simulink model "OcularMotorLabModel_2023_12_21_M21b"  (R2021b)
settings: Solver=FixedStepAuto  StartTime=tStart  StopTime=tFinal  FixedStep=0.001  RelTol=1e-3
undefined symbols (not defined in the file or in its folder): Asp, Asp1, Asp2, e0sp, gaussian, Gpc, GPos, Gsl, HeadToEye, IPD, psi, Psp1, RotFbk, SacThDeg, SatSp, sigbuilder_block, SomFbk, T1, T2, Tccanal, Tcn, Tcr, Tcsp, TCvs, tdm, tdsp1, tdsp2, tdsp3, tdv, Tsl, Tz, w
libraries: matrix_library x16, vrlib x9, simulink_extras x8, simulink x1
(part 1 of 2)
settings Model: Creator=raulr  LastModifiedBy=jom

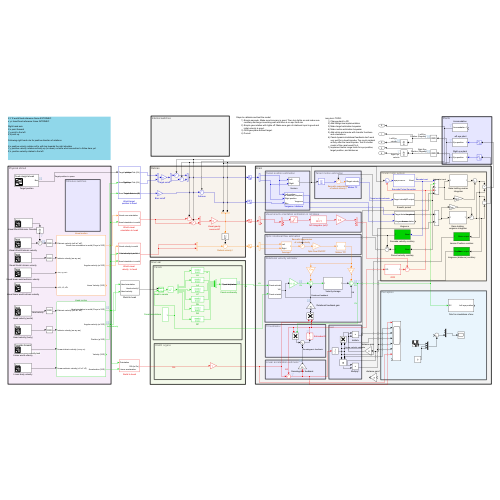
[thumbnail: Simulink's stored preview of the top-level diagram]
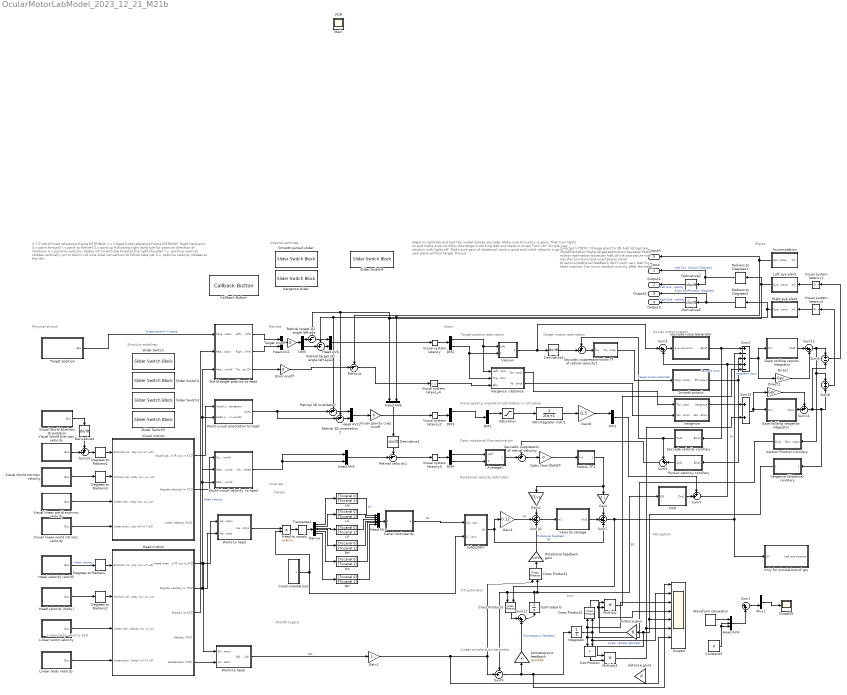
== system OcularMotorLabModel_2023_12_21_M21b ==
  note: Linear body velocity bad
  note: Internal switches
  note: Stimulus switches
  note: Plants
  note: Steps to calibrate and test the model
      | Simple saccade. Make sure Accuracy is good. Then turn lights on and make sure corollary discharge is working well and there is no spv from okn
      | Simple yaw rotation with lights off. Make sure gain of rotational input is good and initial velocity is good.
      | OKN yaw plane without target.
      | Pursuit
  note: X Y Z world fixed reference frame EXTRINSIC
      | x y z head fixed reference frame INTRINSIC
      |
      | Right hand axis
      | X,x point forward
      | Y,y point to the left
      | Z,z point up
      |
      | Following right hand rule for positive direction of rotations
      |
      | X,x positive velocity rotates roll to with top towards the right shoulder
      | Y,y, positive velocity rotates vertically up (or down) not sure what convention to follow here yet
      | Z,z, positive velocity rotates to the left
  note: Brain
  note: Ocular motor system
  note: Perception
  note: Optic rotational flow estimation
  note: Rotational velocity estimator
  note: Linear acceleration estimator
  note: Tilt estimator
  note: Retinas
  note: Otolith organs
  note: Canals
  note: Inner ear
  note: Physical stimuli
  note: Visual gravity orientation estimation in roll plane
  note: Target motion estimation
  note: Target position estimation
  note: tvor
  note: Long term TODO:
      | Change plant to 3D
      | Add listings law implementation
      | Make target estimation bayesian
      | Make motion estimation bayesian
      | Add utricle and sacule with transfer functions and orientations
      | Canal dynamics/rotational feedback don't work very well for a head impulse. Too much residual activity after the head impulse. Test if a better model of the canal would fix it.
      | Implement better range limits for eye position, target position, and distances
  Accomodation : Subsystem
  Average1 : Subsystem
  Blurr on/off : Gain  Gain=0
  Callback Button : CallbackButton  PressDelay=500  RepeatInterval=0  ButtonText=Click to initialize
      settings: ClickFcn=|
      | %% Set parameters
      | tStart = 0;
      | tFinal = 60;
      | 
      | 
      | %% General
      | tdv = 0.050; % visual latency
      | tdm = 0.030; % Motor latency
      | 
      | 
      | %% plant
      | Tz = 0.08;
      | T1 = 0.3;
      | T2 = 0.01; % 0.012
      | w = 200;
      | psi = 1.2;
      | 
      | 
      | %% Saccade system
      | Gpc = 0.06;     % Gain of conjugate pulse
      | Gsl = 0.165;    % Gain of slide
      | Tsl = Tz;     % Tc slide
      | Tcn = 20;       % Tc conjugate neural integrator
      | Tcr = Tcn;       % Tc conjugate resettable integrator
      | 
      | Tep = 0.003;    % Tc motor error pole
      | DelC = 0.006;   % Saccade local feedback delay
      | e0 = 5;
      | AL = 440;
      | AR = 440;
      | lL = 10;
      | LR = 10;
      | SacThDeg = 0.2; % deg
      | 
      | %% Smooth pursuit
      | tdsp1 = 0.015;
      | tdsp2 = 0.035;
      | tdsp3 = 0.030;
      | 
      | Tcsp = 0.007;
      | e0sp = 4;
      | Asp1 = 10;
      | Asp2 = 5;
      | Asp = 1.1;
      | Psp1 = 0.95;
      | Tcsp2 = 0.015;
      | SatSp = 90;
      | 
      | %% Vestibular system
      | Tccanal = 5;
      | TCvs = 11.5;
      | RotFbk = 0.38;
      | SomFbk = 0.65;
      | 
      | %% Integrator
      | GPos = 0.02;
      | 
      | %% Other
      | IPD = 0.06;
      | HeadToEye = 0.05;
      | 
      | 
      | %% simulink initialization
      | signalbuilder([gcs '/Target position'],'activegroup',1)
      | signalbuilder([gcs '/Visual World Extrinsic Orientation'],'activegroup',1)
      | signalbuilder([gcs '/Visual World Extrinsic velocity'],'activegroup',1)
      | signalbuilder([gcs '/Visual World Intrinsic velocity'],'activegroup',1)
      | signalbuilder([gcs '/Visual linear world extrinsic velocity'],'activegroup',1)
      | signalbuilder([gcs '/Visual linear world intrinsic velocity'],'activegroup',1)
      | signalbuilder([gcs '/Head velocity (world)'],'activegroup',1)
      | signalbuilder([gcs '/Head velocity (body)'],'activegroup',1)
      | signalbuilder([gcs '/Linear world velocity'],'activegroup',1)
      | signalbuilder([gcs '/Linear body velocity'],'activegroup',1)
  Canal nonlinearity : Subsystem
  Canal orientations : Subsystem
      settings: PortSchema="{\"entries\":[{\"content\":{\"sides\":[{\"content\":{},\"type\":\"ConnectorPlacement.EquallySpacedRectSide\",\"uuid\":\"1890fa1c-a731-4097-a50e-c33b4fdeb748\"},{\"content\":{\"side\":\"RIGHT\"},\"type\":\"ConnectorPlacement.EquallySpacedRectSide\",\"uuid\":\"2c3145cb-6e74-4844-a72b-94f1b05b1506\"},{\"content\":{\"connectorIds\":[\"Out1\"],\"side\":\"TOP\"},\"type\":\"ConnectorPlacement.EquallySpacedRectSide\",\"uuid\":\"fc07cba5-d6ea-4677-bade-4c6849e180a0\"}]},\"type\":\"ConnectorPlacement.EquallySpacedConnector\",\"uuid\":\"12393832-c76e-4990-8b3e-fdad21d8dbc7\"}],\"packageUris\":[\"http://schema.mathworks.com/mf0/Connector/R2020b\"],\"version\":\"1.0\"}"
  Constant3 : Constant  Value=0
  Cross Product1 : vrlib/Utilities/Cross Product
  Cross Product2 : vrlib/Utilities/Cross Product
  Cross Product3 : vrlib/Utilities/Cross Product
  DM1 : Demux  Outputs=3
  DM{2..5} (4 alike) : Demux  Outputs=2
  Defocus : Sum  Inputs=-+|
  Degrees to Radians{,1..3} (4 alike) : simulink_extras/Transformations/Degrees to Radians
  Demux : Demux  Outputs=6
  Derivative{1..5} (5 alike) : Derivative
  Direct : Gain  Gain=Gpc
  Direct1 : Gain  Gain=Gpc
  Dot Product : DotProduct  InputSameDT=on  OutDataTypeStr=Inherit: Inherit via internal rule
  Estimated G : Integrator  InitialCondition=[0 0 -1]'
  Gain : Gain  Gain=0.1
  Gain1 : Gain
  Gain2 : Gain  Gain=TCvs
  Gain3 : Gain  Gain=0.12
  Gain8 : Gain  Gain=0.5
  Gaze holding vergence integrator : Subsystem
  Gaze holding version Integrator : Subsystem
  Head AV1 : Mux  Inputs=6
  Head AV{2,6,8..9,11} (5 alike) : Mux  Inputs=2
  Head AV4 : Mux  Inputs=3
  Head motion : Subsystem
  Head to canals : Product  Multiplication=Matrix(*)
  Head velocity (body) : Subsystem  Tag=STV Subsys  LoadFcn=sigbuilder_block('load');  StartFcn=sigbuilder_block('start');  StopFcn=sigbuilder_block('stop');  ClipboardFcn=sigbuilder_block('clipboard');  mask(Sigbuilder block){tuvar=[0:10]}
      mask help: Simulink:masks:SigbuilderBlock_MD
      mask init:
      | if ~strcmp(get_param(bdroot(gcbh),'SimulationStatus'),'stopped') tuvar = sigbuilder_block('maskInit'); end
      settings: CopyFcn=sigbuilder_block('copy');  DeleteFcn=sigbuilder_block('delete');  ModelCloseFcn=sigbuilder_block('modelClose');  PreSaveFcn=sigbuilder_block('preSave');  PauseFcn=sigbuilder_block('pause');  ContinueFcn=sigbuilder_block('continue');  NameChangeFcn=sigbuilder_block('namechange');  OpenFcn=sigbuilder_block('open',[773.5 227.4 1141 504.1 ]);  CloseFcn=sigbuilder_block('close');
      mask Display: plot(0, 0, 100, 100,[2, 2, 32, 32, 2], [68, 8, 8, 68, 68],[32, 2], [38, 38], [32, 19, 2],[53, 60, 44], [32, 17, 17, 2],[16, 16, 31, 31]);txt = getActiveGroup(gcbh);text(2, 100, txt,'verticalAlignment', 'top');
  Head velocity (world) : Subsystem  Tag=STV Subsys  LoadFcn=sigbuilder_block('load');  StartFcn=sigbuilder_block('start');  StopFcn=sigbuilder_block('stop');  ClipboardFcn=sigbuilder_block('clipboard');  mask(Sigbuilder block){tuvar=[0:10]}
      mask help: Simulink:masks:SigbuilderBlock_MD
      mask init:
      | if ~strcmp(get_param(bdroot(gcbh),'SimulationStatus'),'stopped') tuvar = sigbuilder_block('maskInit'); end
      settings: CopyFcn=sigbuilder_block('copy');  DeleteFcn=sigbuilder_block('delete');  ModelCloseFcn=sigbuilder_block('modelClose');  PreSaveFcn=sigbuilder_block('preSave');  PauseFcn=sigbuilder_block('pause');  ContinueFcn=sigbuilder_block('continue');  NameChangeFcn=sigbuilder_block('namechange');  OpenFcn=sigbuilder_block('open',[555 156 1141.2 654.6 ]);  CloseFcn=sigbuilder_block('close');
      mask Display: plot(0, 0, 100, 100,[2, 2, 32, 32, 2], [68, 8, 8, 68, 68],[32, 2], [38, 38], [32, 19, 2],[53, 60, 44], [32, 17, 17, 2],[16, 16, 31, 31]);txt = getActiveGroup(gcbh);text(2, 100, txt,'verticalAlignment', 'top');
  Integrator : Integrator
  LA : TransferFcn  Numerator=[Tccanal 0]  Denominator=[Tccanal 1]
  LH : TransferFcn  Numerator=[Tccanal 0]  Denominator=[Tccanal 1]
  LP : TransferFcn  Numerator=[Tccanal 0]  Denominator=[Tccanal 1]
  Left eye plant : Subsystem
  Linear body velocity : Subsystem  Tag=STV Subsys  LoadFcn=sigbuilder_block('load');  StartFcn=sigbuilder_block('start');  StopFcn=sigbuilder_block('stop');  ClipboardFcn=sigbuilder_block('clipboard');  mask(Sigbuilder block){tuvar=[0:10]}
      mask help: Simulink:masks:SigbuilderBlock_MD
      mask init:
      | if ~strcmp(get_param(bdroot(gcbh),'SimulationStatus'),'stopped') tuvar = sigbuilder_block('maskInit'); end
      settings: CopyFcn=sigbuilder_block('copy');  DeleteFcn=sigbuilder_block('delete');  ModelCloseFcn=sigbuilder_block('modelClose');  PreSaveFcn=sigbuilder_block('preSave');  PauseFcn=sigbuilder_block('pause');  ContinueFcn=sigbuilder_block('continue');  NameChangeFcn=sigbuilder_block('namechange');  OpenFcn=sigbuilder_block('open',[773.5 227.4 1141 504.1 ]);  CloseFcn=sigbuilder_block('close');
      mask Display: plot(0, 0, 100, 100,[2, 2, 32, 32, 2], [68, 8, 8, 68, 68],[32, 2], [38, 38], [32, 19, 2],[53, 60, 44], [32, 17, 17, 2],[16, 16, 31, 31]);txt = getActiveGroup(gcbh);text(2, 100, txt,'verticalAlignment', 'top');
  Linear world velocity : Subsystem  Tag=STV Subsys  LoadFcn=sigbuilder_block('load');  StartFcn=sigbuilder_block('start');  StopFcn=sigbuilder_block('stop');  ClipboardFcn=sigbuilder_block('clipboard');  mask(Sigbuilder block){tuvar=[0:10]}
      mask help: Simulink:masks:SigbuilderBlock_MD
      mask init:
      | if ~strcmp(get_param(bdroot(gcbh),'SimulationStatus'),'stopped') tuvar = sigbuilder_block('maskInit'); end
      settings: CopyFcn=sigbuilder_block('copy');  DeleteFcn=sigbuilder_block('delete');  ModelCloseFcn=sigbuilder_block('modelClose');  PreSaveFcn=sigbuilder_block('preSave');  PauseFcn=sigbuilder_block('pause');  ContinueFcn=sigbuilder_block('continue');  NameChangeFcn=sigbuilder_block('namechange');  OpenFcn=sigbuilder_block('open',[773.5 227.4 1141 504.1 ]);  CloseFcn=sigbuilder_block('close');
      mask Display: plot(0, 0, 100, 100,[2, 2, 32, 32, 2], [68, 8, 8, 68, 68],[32, 2], [38, 38], [32, 19, 2],[53, 60, 44], [32, 17, 17, 2],[16, 16, 31, 31]);txt = getActiveGroup(gcbh);text(2, 100, txt,'verticalAlignment', 'top');
  MX1 : Mux  Inputs=3
  Motion TF : Subsystem
  Motion TF1 : Subsystem
  Multiply : Product  Inputs=**
  Multiply1 : Product  Inputs=**
  Mux1 : Mux  Inputs=2
  NO Integrator (roll)1 : TransferFcn  Denominator=[20 1]
  OCR : Subsystem
  Only for simulations of spv : Subsystem
  Optic flow ON/OFF : Gain  Gain=0
  Pursuit velocity corollary : Subsystem
  RA : TransferFcn  Numerator=[Tccanal 0]  Denominator=[Tccanal 1]
  RH : TransferFcn  Numerator=[Tccanal 0]  Denominator=[Tccanal 1]
  RP : TransferFcn  Numerator=[Tccanal 0]  Denominator=[Tccanal 1]
  Radians to Degrees1 : simulink_extras/Transformations/Radians to Degrees
  Radians to Degrees2 : simulink_extras/Transformations/Radians to Degrees
  Retinal 3D orientation : Sum  Inputs=++|
  Retinal 3D orientation1 : Sum  Inputs=++|
  Retinal target 2D angle left eye : Sum  Inputs=-+|
  Retinal target 2D angle left eye1 : Sum  Inputs=-+|
  Retinal velocity1 : Sum  Inputs=-+|
  Right eye plant : Subsystem
  Rotational feedback gain : Gain  Gain=RotFbk
  Saccade Pulse Generator : Subsystem
  Saccade velocity corollary : Subsystem
  Saccadic suppression of retinal velocity : Sum  Inputs=++|
  Saccadic suppression of retinal velocity1 : Sum  Inputs=++|
  Saturation : Saturate  UpperLimit=5*pi/180  LowerLimit=-5*pi/180
  Scope29 : Scope
  Scope3 : Scope  NumInputPorts=8
  Slider Switch{,1..4} (5 alike) : SliderSwitchBlock
      settings: Values={{'Off', 'On'}, [0 1]}
  Smooth pursuit : Subsystem
  Smooth pursuit slider : SliderSwitchBlock
      settings: Values={{'Off', 'On'}, [0 1]}
  Somatogravic feedback : Gain  Gain=SomFbk
  Subsystem : Subsystem
  Sum{1,3,11..12} (4 alike) : Sum  Inputs=|++
  Sum10 : Sum  Inputs=+++
  Sum{4,6,13..14} (4 alike) : Sum  Inputs=++|
  Sum15 : Sum
  Sum2 : Sum  Inputs=+-++-
  Sum5 : Sum  Inputs=+-
  Sum7 : Sum  Inputs=+++
  Sum8 : Sum  Inputs=+|+
  Sum9 : Sum  Inputs=-+|
  Target on/off : Gain  Gain=0
  Target position : Subsystem  Tag=STV Subsys  LoadFcn=sigbuilder_block('load');  StartFcn=sigbuilder_block('start');  StopFcn=sigbuilder_block('stop');  ClipboardFcn=sigbuilder_block('clipboard');  mask(Sigbuilder block){tuvar=[0:10]}
      mask help: Simulink:masks:SigbuilderBlock_MD
      mask init:
      | if ~strcmp(get_param(bdroot(gcbh),'SimulationStatus'),'stopped') tuvar = sigbuilder_block('maskInit'); end
      settings: CopyFcn=sigbuilder_block('copy');  DeleteFcn=sigbuilder_block('delete');  ModelCloseFcn=sigbuilder_block('modelClose');  PreSaveFcn=sigbuilder_block('preSave');  PauseFcn=sigbuilder_block('pause');  ContinueFcn=sigbuilder_block('continue');  NameChangeFcn=sigbuilder_block('namechange');  OpenFcn=sigbuilder_block('open',[653.4 220.2 1116.6 655.8 ]);  CloseFcn=sigbuilder_block('close');
      mask Display: plot(0, 0, 100, 100,[2, 2, 32, 32, 2], [68, 8, 8, 68, 68],[32, 2], [38, 38], [32, 19, 2],[53, 60, 44], [32, 17, 17, 2],[16, 16, 31, 31]);txt = getActiveGroup(gcbh);text(2, 100, txt,'verticalAlignment', 'top');
  Transpose1 : matrix_library/Transpose
  Velocity storage : Subsystem
  Vergence : Subsystem
  Vergence (distance) corollary : Subsystem
  Vergence / distance : Subsystem
  Vergence slider : SliderSwitchBlock
      settings: Values={{'Off', 'On'}, [0 1]}
  Version : Subsystem
  Version Position corollary : Subsystem
  Visual World Extrinsic Orientation : Subsystem  Tag=STV Subsys  LoadFcn=sigbuilder_block('load');  StartFcn=sigbuilder_block('start');  StopFcn=sigbuilder_block('stop');  ClipboardFcn=sigbuilder_block('clipboard');  mask(Sigbuilder block){tuvar=[0:10]}
      mask help: Simulink:masks:SigbuilderBlock_MD
      mask init:
      | if ~strcmp(get_param(bdroot(gcbh),'SimulationStatus'),'stopped') tuvar = sigbuilder_block('maskInit'); end
      settings: CopyFcn=sigbuilder_block('copy');  DeleteFcn=sigbuilder_block('delete');  ModelCloseFcn=sigbuilder_block('modelClose');  PreSaveFcn=sigbuilder_block('preSave');  PauseFcn=sigbuilder_block('pause');  ContinueFcn=sigbuilder_block('continue');  NameChangeFcn=sigbuilder_block('namechange');  OpenFcn=sigbuilder_block('open',[244.2 225.6 1909.2 712.8 ]);  CloseFcn=sigbuilder_block('close');
      mask Display: plot(0, 0, 100, 100,[2, 2, 32, 32, 2], [68, 8, 8, 68, 68],[32, 2], [38, 38], [32, 19, 2],[53, 60, 44], [32, 17, 17, 2],[16, 16, 31, 31]);txt = getActiveGroup(gcbh);text(2, 100, txt,'verticalAlignment', 'top');
  Visual World Extrinsic velocity : Subsystem  Tag=STV Subsys  LoadFcn=sigbuilder_block('load');  StartFcn=sigbuilder_block('start');  StopFcn=sigbuilder_block('stop');  ClipboardFcn=sigbuilder_block('clipboard');  mask(Sigbuilder block){tuvar=[0:10]}
      mask help: Simulink:masks:SigbuilderBlock_MD
      mask init:
      | if ~strcmp(get_param(bdroot(gcbh),'SimulationStatus'),'stopped') tuvar = sigbuilder_block('maskInit'); end
      settings: CopyFcn=sigbuilder_block('copy');  DeleteFcn=sigbuilder_block('delete');  ModelCloseFcn=sigbuilder_block('modelClose');  PreSaveFcn=sigbuilder_block('preSave');  PauseFcn=sigbuilder_block('pause');  ContinueFcn=sigbuilder_block('continue');  NameChangeFcn=sigbuilder_block('namechange');  OpenFcn=sigbuilder_block('open',[5.5 135 1909 675.5 ]);  CloseFcn=sigbuilder_block('close');
      mask Display: plot(0, 0, 100, 100,[2, 2, 32, 32, 2], [68, 8, 8, 68, 68],[32, 2], [38, 38], [32, 19, 2],[53, 60, 44], [32, 17, 17, 2],[16, 16, 31, 31]);txt = getActiveGroup(gcbh);text(2, 100, txt,'verticalAlignment', 'top');
  Visual World Intrinsic velocity : Subsystem  Tag=STV Subsys  LoadFcn=sigbuilder_block('load');  StartFcn=sigbuilder_block('start');  StopFcn=sigbuilder_block('stop');  ClipboardFcn=sigbuilder_block('clipboard');  mask(Sigbuilder block){tuvar=[0:10]}
      mask help: Simulink:masks:SigbuilderBlock_MD
      mask init:
      | if ~strcmp(get_param(bdroot(gcbh),'SimulationStatus'),'stopped') tuvar = sigbuilder_block('maskInit'); end
      settings: CopyFcn=sigbuilder_block('copy');  DeleteFcn=sigbuilder_block('delete');  ModelCloseFcn=sigbuilder_block('modelClose');  PreSaveFcn=sigbuilder_block('preSave');  PauseFcn=sigbuilder_block('pause');  ContinueFcn=sigbuilder_block('continue');  NameChangeFcn=sigbuilder_block('namechange');  OpenFcn=sigbuilder_block('open',[5.5 135 1909 675.5 ]);  CloseFcn=sigbuilder_block('close');
      mask Display: plot(0, 0, 100, 100,[2, 2, 32, 32, 2], [68, 8, 8, 68, 68],[32, 2], [38, 38], [32, 19, 2],[53, 60, 44], [32, 17, 17, 2],[16, 16, 31, 31]);txt = getActiveGroup(gcbh);text(2, 100, txt,'verticalAlignment', 'top');
  Visual gravity cues on/off : Gain  Gain=0
  Visual linear world extrinsic velocity : Subsystem  Tag=STV Subsys  LoadFcn=sigbuilder_block('load');  StartFcn=sigbuilder_block('start');  StopFcn=sigbuilder_block('stop');  ClipboardFcn=sigbuilder_block('clipboard');  mask(Sigbuilder block){tuvar=[0:10]}
      mask help: Simulink:masks:SigbuilderBlock_MD
      mask init:
      | if ~strcmp(get_param(bdroot(gcbh),'SimulationStatus'),'stopped') tuvar = sigbuilder_block('maskInit'); end
      settings: CopyFcn=sigbuilder_block('copy');  DeleteFcn=sigbuilder_block('delete');  ModelCloseFcn=sigbuilder_block('modelClose');  PreSaveFcn=sigbuilder_block('preSave');  PauseFcn=sigbuilder_block('pause');  ContinueFcn=sigbuilder_block('continue');  NameChangeFcn=sigbuilder_block('namechange');  OpenFcn=sigbuilder_block('open',[773.5 227.4 1141 504.1 ]);  CloseFcn=sigbuilder_block('close');
      mask Display: plot(0, 0, 100, 100,[2, 2, 32, 32, 2], [68, 8, 8, 68, 68],[32, 2], [38, 38], [32, 19, 2],[53, 60, 44], [32, 17, 17, 2],[16, 16, 31, 31]);txt = getActiveGroup(gcbh);text(2, 100, txt,'verticalAlignment', 'top');
  Visual linear world intrinsic velocity : Subsystem  Tag=STV Subsys  LoadFcn=sigbuilder_block('load');  StartFcn=sigbuilder_block('start');  StopFcn=sigbuilder_block('stop');  ClipboardFcn=sigbuilder_block('clipboard');  mask(Sigbuilder block){tuvar=[0:10]}
      mask help: Simulink:masks:SigbuilderBlock_MD
      mask init:
      | if ~strcmp(get_param(bdroot(gcbh),'SimulationStatus'),'stopped') tuvar = sigbuilder_block('maskInit'); end
      settings: CopyFcn=sigbuilder_block('copy');  DeleteFcn=sigbuilder_block('delete');  ModelCloseFcn=sigbuilder_block('modelClose');  PreSaveFcn=sigbuilder_block('preSave');  PauseFcn=sigbuilder_block('pause');  ContinueFcn=sigbuilder_block('continue');  NameChangeFcn=sigbuilder_block('namechange');  OpenFcn=sigbuilder_block('open',[773.5 227.4 1141 504.1 ]);  CloseFcn=sigbuilder_block('close');
      mask Display: plot(0, 0, 100, 100,[2, 2, 32, 32, 2], [68, 8, 8, 68, 68],[32, 2], [38, 38], [32, 19, 2],[53, 60, 44], [32, 17, 17, 2],[16, 16, 31, 31]);txt = getActiveGroup(gcbh);text(2, 100, txt,'verticalAlignment', 'top');
  Visual motion : Subsystem
  Visual system latency{,2..4} (4 alike) : TransportDelay  DelayTime=tdv
  Visual system latency1 : TransportDelay  DelayTime=tdm
  Visual system latency5 : TransportDelay  DelayTime=tdm
  Waveform Generator : simulink/Sources/Waveform Generator  OutMin=[]  OutMax=[]  OutDataTypeStr=double  SelectedSignal=1  Signals=gaussian(0,0.1,1)  BlockNames=MultiportSwitch_125da93d47db44d  SampleTime=0.1
  World target position to head : Subsystem
  World to head : Subsystem
  "World to head " : Subsystem
  World visual orientation to head : Subsystem
  World visual velocity  to head : Subsystem
  distance gain : Gain  Gain=8
  distance gain1 : Gain  Gain=8
  Output : Outport
  Output1 : Outport  Port=2
  Output2 : Outport  Port=3
  Output3 : Outport  Port=4
  Output4 : Outport  Port=5
  Main : Scope
  VOR : Scope
  wires:
  Sum7/1 -> Only for simulations of spv/1(EV), Sum2/2, Cross Product3/2  "EV"
  Sum9/1 -> Scope3/1, Integrator/1, Somatogravic feedback/1
  Cross Product3/1 -> Sum11/1
  Estimated G/1 -> Cross Product1/2, OCR/1(EG), Sum9/1, Cross Product3/1  "EG"
  Cross Product1/1 -> Rotational feedback gain/1
  Head velocity (world)/1(Bus) -> Degrees to Radians/1  "Head velocity"
  Sum11/1 -> Estimated G/1
  Rotational feedback gain/1 -> Sum10/3  "Rotational feedback"
  Somatogravic feedback/1 -> Sum11/2  "Somatogravic feedback"
  Gain1/1 -> Scope3/7, Sum9/2, Cross Product1/1
  Gain3/1 -> Sum10/2  "VN"
  Motion TF1/1(Out1) -> Gain2/1, Gain/1
  Gain/1 -> Sum7/1
  Radians to Degrees1/1 -> Derivative2/1, Output/1  "Left Eye  Position (Degrees)"
  NO Integrator (roll)1/1 -> Gain8/1
  MX1/1 -> Sum4/1
  Sum1/1 -> Mux1/2
  Mux1/1 -> Scope29/1
  Constant3/1 -> Head AV4/2, Head AV4/3
  Waveform Generator/1 -> Head AV4/1
  Head AV4/1 -> Sum1/2
  Saccade Pulse Generator/1(Burst) -> Saccade velocity corollary/1(Burst), Sum2/1  "Saccade burst"
  Sum2/1 -> Direct/1, Gaze holding version Integrator/1(In1)  "Integrator input"
  Optic flow ON/OFF/1 -> Motion TF1/1(In1)
  Saccadic suppression of retinal velocity/1 -> Optic flow ON/OFF/1
  Sum4/1 -> Sum3/2, Sum2/4
  Head velocity (body)/1(Bus) -> Degrees to Radians2/1
  Degrees to Radians2/1 -> Head motion/2(Intrinsic velocity (wx wy wz))
  Degrees to Radians/1 -> Head motion/1(Extrinsic velocity (wX wY wZ))
  Head motion/1(Head orientation in world (R xyz in XYZ)) -> World to head/1(Orientation), "World to head "/1(Head orientation), World target position to head/3(Head orientation in world), World visual orientation to head/2(Head orientation in world1), World visual velocity  to head/3(Head orientation in world)
  Head motion/5(Acceleration (XYZ)) -> World to head/2(Linear acceleration)
  Head motion/2(Angular velocity (w XYZ)) -> World visual velocity  to head/2(Head velocity in world), "World to head "/2(Head velocity)  "Head velocity"
  Degrees to Radians1/1 -> Visual motion/1(Extrinsic velocity (wX wY wZ))
  Target position/1(Bus) -> World target position to head/1(Target position)  "Target position in space"
  Head motion/3(Position (p XYZ)) -> World target position to head/2(Head position)
  Visual motion/1(Visual cues orientation in world (R xyz in XYZ)) -> World visual orientation to head/1(Visual cues orientation)
  Visual motion/2(Angular velocity (w XYZ)) -> World visual velocity  to head/1(Visual velocity in world)
  World visual velocity  to head/1(Visual velocity in Head) -> Head AV9/1, Head AV9/2
  Head to canals/1 -> Transpose1/1
  World target position to head/1(Left eye Fick (HV)) -> Head AV2/1
  World to head/1(GIA (in Gs)) -> Gain1/1  "GIA"
  Sum3/1 -> Saccade Pulse Generator/1(eye pos error)
  OCR/1(Out1) -> Sum4/2
  Saturation/1 -> NO Integrator (roll)1/1
  DM1/1 -> Saturation/1
  Gain8/1 -> MX1/1
  Version/1(Out1) -> Derivative3/1, Sum3/1
  Motion TF/1(Target velocity) -> Smooth pursuit/1(Target velocity)  "Target motion estimate"
  DM2/1 -> Vergence / distance/1(Left position), Version/1(Left)
  DM3/1 -> DM1/1
  Retinal velocity1/1 -> Visual system latency3/1
  Gain2/1 -> Sum10/1
  Derivative1/1 -> Retinal velocity1/1
  Visual system latency3/1 -> DM4/1
  Saccade velocity corollary/1(Out1) -> Saccadic suppression of retinal velocity1/1, Sum6/1
  Smooth pursuit/1(SP output) -> Pursuit velocity corollary/1(Burst), Sum2/3
  World target position to head/3(Target distance (D)) -> Blurr on/off/1
  Defocus/1 -> Visual system latency4/1
  Head AV6/1 -> Visual system latency/1
  DM2/2 -> Vergence / distance/2(Right position), Version/2(Right)
  Visual system latency4/1 -> Vergence / distance/3(Blur)
  Average1/1(Out1) -> Saccadic suppression of retinal velocity/2
  DM4/2 -> Average1/2(Right)
  Visual system latency/1 -> DM2/1
  Visual system latency2/1 -> DM3/1
  Head AV8/1 -> Derivative1/1
  DM4/1 -> Average1/1(Left)
  Head AV9/1 -> Retinal velocity1/2
  DM5/1 -> Retinal target 2D angle left eye/2
  World visual orientation to head/1(Out1) -> Retinal 3D orientation/2, Retinal 3D orientation1/2
  Retinal target 2D angle left eye/1 -> Head AV6/1
  Retinal target 2D angle left eye1/1 -> Head AV6/2
  Derivative3/1 -> Saccadic suppression of retinal velocity1/2
  Saccadic suppression of retinal velocity1/1 -> Motion TF/1(In1)
  Sum6/1 -> Saccadic suppression of retinal velocity/1
  Pursuit velocity corollary/1(Out1) -> Sum6/2
  Right eye plant/1(Eye position) -> Radians to Degrees2/1, Retinal target 2D angle left eye1/1, Retinal 3D orientation/1, Head AV8/2
  Accomodation/1(Accomodation) -> Output4/1, Defocus/1
  Sum5/1 -> Visual system latency1/1
  Left eye plant/1(Eye position) -> Radians to Degrees1/1, Retinal target 2D angle left eye/1, Retinal 3D orientation1/1, Head AV8/1
  Blurr on/off/1 -> Defocus/2
  Retinal 3D orientation1/1 -> Head AV11/2
  Retinal 3D orientation/1 -> Head AV11/1
  Head AV11/1 -> Visual gravity cues on/off/1
  Sum15/1 -> Direct1/1, Gaze holding vergence integrator/1(In1)
  Direct/1 -> Sum12/2
  Visual system latency1/1 -> Left eye plant/1(In1)
  Visual system latency5/1 -> Right eye plant/1(In1)
  Sum10/1 -> Velocity storage/1(In1)
  Velocity storage/1(Out1) -> Sum7/2
  Visual gravity cues on/off/1 -> Visual system latency2/1
  Derivative2/1 -> Output1/1  "Left Eye  velocity"
  Derivative5/1 -> Output3/1  "Right Eye  velocity"
  Radians to Degrees2/1 -> Output2/1, Derivative5/1  "Right Eye  Position (Degrees)"
  Visual World Extrinsic Orientation/1(Bus) -> Derivative4/1
  Sum13/1 -> Degrees to Radians1/1
  Derivative4/1 -> Sum13/1
  Visual World Extrinsic velocity/1(Bus) -> Sum13/2
  Integrator/1 -> Dot Product/2, Scope3/2, Cross Product2/2  "Linear velocity estimate"
  Dot Product/1 -> Multiply1/2
  "World to head "/1(Head velocity1) -> Head to canals/1
  World target position to head/2(Right eye Fick (HV)) -> Head AV2/2
  Head AV2/1 -> Target on/off/1
  DM5/2 -> Retinal target 2D angle left eye1/2
  Target on/off/1 -> DM5/1
  Degrees to Radians3/1 -> Visual motion/2(Intrinsic velocity (wx wy wz))
  Visual World Intrinsic velocity/1(Bus) -> Degrees to Radians3/1
  distance gain/1 -> Multiply/1
  Gaze holding version Integrator/1(Out1) -> Sum12/1
  Sum12/1 -> Sum5/1, Version Position corollary/1(Motor output), Sum8/1
  Gaze holding vergence integrator/1(Out1) -> Sum14/2
  Sum8/1 -> Visual system latency5/1
  Direct1/1 -> Sum14/1
  Sum14/1 -> Vergence (distance) corollary/1(Motor output), Sum8/2, Sum5/2
  Vergence / distance/2(Vergence) -> Vergence/2(Vergence error)
  Vergence / distance/1(Target distance estimate (Diopters)) -> Vergence/1(Target distance estimate (Diopters))
  Linear world velocity/1(Bus) -> Head motion/3(Linear intrinsic velocity (vx vy vz))
  Version Position corollary/1(Out1) -> Dot Product/1, Scope3/3, Cross Product2/1
  Cross Product2/1 -> Scope3/4, Multiply/2
  Vergence/1(Vergence) -> Sum15/1
  Linear body velocity/1(Bus) -> Head motion/4(Linear extrinsic velocity (vX vY vZ))
  Visual linear world extrinsic velocity/1(Bus) -> Visual motion/3(Linear intrinsic velocity (wx wy wz))
  Visual linear world intrinsic velocity/1(Bus) -> Visual motion/4(Linear extrinsic velocity (wX wY wZ))
  Canal orientations/1(Out1) -> Subsystem/2(Canal orientations), Head to canals/2
  Demux/2 -> LA/1
  RH/1 -> Head AV1/4
  LH/1 -> Head AV1/1  "LH"
  LP/1 -> Head AV1/3
  Demux/4 -> RH/1
  RP/1 -> Head AV1/6
  Demux/6 -> RP/1
  RA/1 -> Head AV1/5
  Demux/5 -> RA/1
  Demux/1 -> LH/1
  LA/1 -> Head AV1/2
  Demux/3 -> LP/1
  Transpose1/1 -> Demux/1
  Head AV1/1 -> Canal nonlinearity/1(Cupula displacement)
  Canal nonlinearity/1(Canal activation) -> Subsystem/1(Canal activation)  "VN"
  Subsystem/1(VN) -> Sum7/3, Gain3/1  "VN"
  Multiply/1 -> Sum2/5
  Vergence (distance) corollary/1(Diopters) -> Scope3/5, Multiply1/1, distance gain/1
  Multiply1/1 -> Scope3/6, Sum15/2

== system OcularMotorLabModel_2023_12_21_M21b/Accomodation ==
  In1 : Inport
  Accomodation : Outport

== system OcularMotorLabModel_2023_12_21_M21b/Average1 ==
  Left : Inport
  Right : Inport  Port=2
  Constant : Constant  Value=2
  Divide : Product  Inputs=*/
  Sum : Sum  Inputs=|++
  Out1 : Outport
  wires:
  Divide/1 -> Out1/1
  Sum/1 -> Divide/1
  Left/1 -> Sum/1
  Constant/1 -> Divide/2
  Right/1 -> Sum/2

== system OcularMotorLabModel_2023_12_21_M21b/Canal nonlinearity ==
  note: Nonlinearity of the canals
      |
      | Baseline firing rate corresponding to a speed of 100 deg/s
      |
      | No negative respose
      |
      | To correctly average both sides and get a continuos linear slope. We need to have a piecewise gain that is half during the bilateral range [-100 to 100]
  Cupula displacement : Inport
  Baseline rate : Constant  Value=100
  Gain : Gain  Gain=1/2
  Radians to Degrees : simulink_extras/Transformations/Radians to Degrees
  Saturation : Saturate  UpperLimit=100  LowerLimit=-100
  Saturation1 : Saturate  UpperLimit=inf  LowerLimit=0
  Sum1 : Sum  Inputs=++-
  Canal activation : Outport
  wires:
  Saturation1/1 -> Canal activation/1
  Sum1/1 -> Saturation1/1
  Saturation/1 -> Gain/1
  Radians to Degrees/1 -> Sum1/2, Saturation/1
  Cupula displacement/1 -> Radians to Degrees/1
  Baseline rate/1 -> Sum1/1
  Gain/1 -> Sum1/3

== system OcularMotorLabModel_2023_12_21_M21b/Canal orientations ==
  note: https://www.ncbi.nlm.nih.gov/pmc/articles/PMC2504595/
  Canal orientations LHLALPRHRARP : Constant  Value=|  VectorParams1D=off
      | [-0.32269 -0.03837 0.94573; -0.5893 0.78839 -0.17655; -0.69432 -0.66693 -0.27042; 
      |     -0.32269 0.03837 0.94573; -0.5893 -0.78839 -0.17655; -0.69432 0.66693 -0.27042]
  Excitation/inhibition : Constant  Value=[ones(3);-ones(3)]  VectorParams1D=off
  Product : Product
  Transpose : matrix_library/Transpose
  Out1 : Outport
  wires:
  Transpose/1 -> Out1/1
  Canal orientations LHLALPRHRARP/1 -> Product/1
  Excitation/inhibition/1 -> Product/2
  Product/1 -> Transpose/1

== system OcularMotorLabModel_2023_12_21_M21b/Gaze holding vergence integrator ==
  In1 : Inport
  Position bias3 : TransferFcn  Numerator=[Tcn]  Denominator=[Tcn 1]
  Sum1 : Sum  Inputs=|++
  Vergence set point : Constant  Value=deg2rad(2)/Tcn
  Out1 : Outport
  wires:
  Position bias3/1 -> Out1/1
  Vergence set point/1 -> Sum1/2
  Sum1/1 -> Position bias3/1
  In1/1 -> Sum1/1

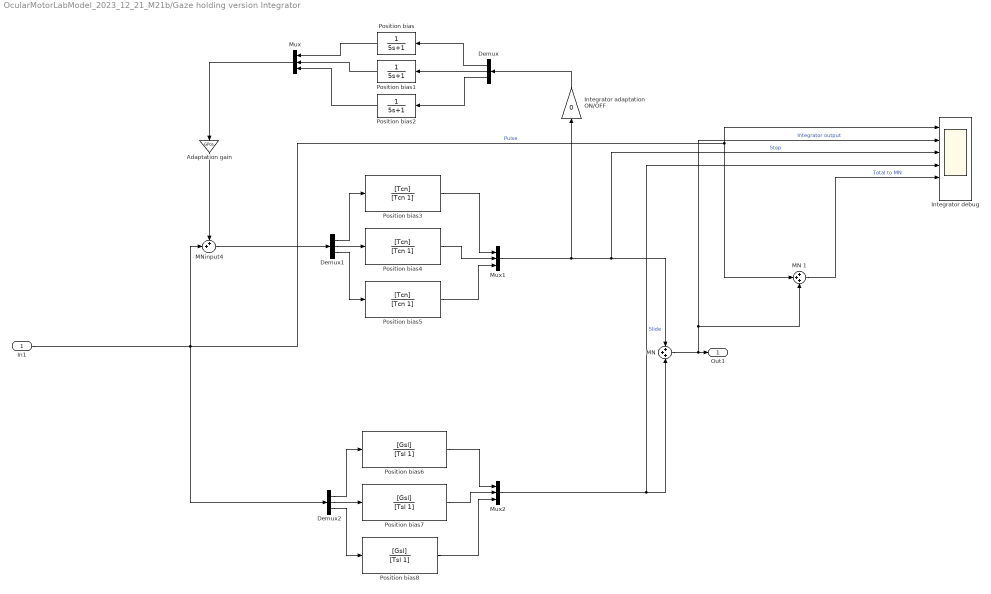
== system OcularMotorLabModel_2023_12_21_M21b/Gaze holding version Integrator ==
  In1 : Inport
  Adaptation gain : Gain  Gain=GPos
  Demux : Demux  Outputs=3
  Demux1 : Demux  Outputs=3
  Demux2 : Demux  Outputs=3
  Integrator adaptation ON/OFF : Gain  Gain=0
  Integrator debug : Scope  NumInputPorts=6
  "MN " : Sum  Inputs=+++  InputSameDT=on  SaturateOnIntegerOverflow=on  OutDataTypeStr=Inherit: Same as first input
  MN 1 : Sum  Inputs=+++  InputSameDT=on  SaturateOnIntegerOverflow=on  OutDataTypeStr=Inherit: Same as first input
  MNinput4 : Sum  Inputs=++|  InputSameDT=on  SaturateOnIntegerOverflow=on  OutDataTypeStr=Inherit: Same as first input
  Mux : Mux  Inputs=3
  Mux1 : Mux  Inputs=3
  Mux2 : Mux  Inputs=3
  Position bias : TransferFcn  Numerator=1  Denominator=[5 1]
  Position bias1 : TransferFcn  Numerator=1  Denominator=[5 1]
  Position bias2 : TransferFcn  Numerator=1  Denominator=[5 1]
  Position bias3 : TransferFcn  Numerator=[Tcn]  Denominator=[Tcn 1]
  Position bias4 : TransferFcn  Numerator=[Tcn]  Denominator=[Tcn 1]
  Position bias5 : TransferFcn  Numerator=[Tcn]  Denominator=[Tcn 1]
  Position bias6 : TransferFcn  Numerator=[Gsl]  Denominator=[Tsl 1]
  Position bias7 : TransferFcn  Numerator=[Gsl]  Denominator=[Tsl 1]
  Position bias8 : TransferFcn  Numerator=[Gsl]  Denominator=[Tsl 1]
  Out1 : Outport
  wires:
  Mux/1 -> Adaptation gain/1
  Demux/1 -> Position bias/1
  Demux/2 -> Position bias1/1
  Demux/3 -> Position bias2/1
  Position bias1/1 -> Mux/2
  Position bias/1 -> Mux/1
  Position bias2/1 -> Mux/3
  MNinput4/1 -> Demux1/1
  Position bias4/1 -> Mux1/2
  Demux1/3 -> Position bias5/1
  Mux1/1 -> Integrator debug/3, "MN "/1, Integrator adaptation ON/OFF/1  "Step"
  Position bias5/1 -> Mux1/3
  Position bias3/1 -> Mux1/1
  Demux1/2 -> Position bias4/1
  Demux1/1 -> Position bias3/1
  Position bias7/1 -> Mux2/2
  In1/1 -> MN 1/2, Integrator debug/1, MNinput4/2, Demux2/1  "Pulse"
  Demux2/1 -> Position bias6/1
  Position bias6/1 -> Mux2/1
  Demux2/3 -> Position bias8/1
  Position bias8/1 -> Mux2/3
  Demux2/2 -> Position bias7/1
  Mux2/1 -> "MN "/3, Integrator debug/4  "Slide"
  "MN "/1 -> MN 1/3, Integrator debug/2, Out1/1  "Integrator output"
  Adaptation gain/1 -> MNinput4/1
  MN 1/1 -> Integrator debug/5  "Total to MN"
  Integrator adaptation ON/OFF/1 -> Demux/1

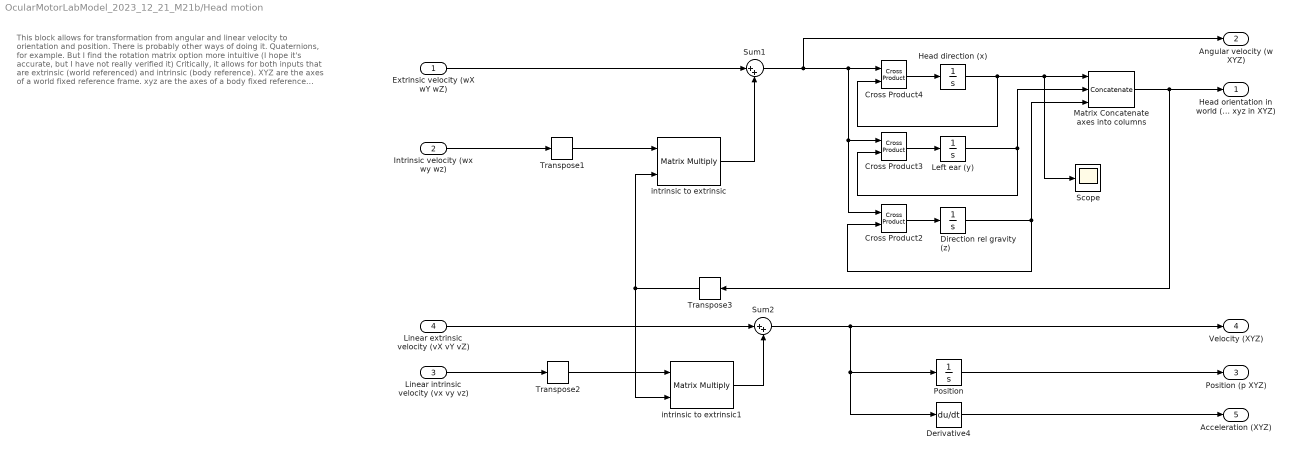
== system OcularMotorLabModel_2023_12_21_M21b/Head motion ==
  note: This block allows for transformation from angular and linear velocity to orientation and position. There is probably other ways of doing it. Quaternions, for example. But I find the rotation matrix option more intuitive (I hope it's accurate, but I have not really verified it)
      |
      | Critically, it allows for both inputs that are extrinsic (world referenced) and intrinsic (body reference).
      |
      | XYZ are the axes of a world fixed reference frame.
      | xyz are the axes of a body fixed reference frame
      |
      | For the extrinsic angular velocities, they need to be integrated after a cross product with each of the xyz axis, that way they provide the rotation of such axis within the XYZ world fixed reference frame.
      |
      | For the intrinsic angular velocities, they simply multiply each of the intrisic axis and get added to the extrinsic velocities.
      |
      | A similar approach is followed for the linear velocities but without the cross products are linear velocities can be simply integrated by components.
  Extrinsic velocity (wX wY wZ) : Inport
  Intrinsic velocity (wx wy wz) : Inport  Port=2
  Linear intrinsic velocity (vx vy vz) : Inport  Port=3
  Linear extrinsic velocity (vX vY vZ) : Inport  Port=4
  Cross Product2 : vrlib/Utilities/Cross Product
  Cross Product3 : vrlib/Utilities/Cross Product
  Cross Product4 : vrlib/Utilities/Cross Product
  Derivative4 : Derivative
  Direction rel gravity (z) : Integrator  InitialCondition=[0 0 1]
  Head direction (x) : Integrator  InitialCondition=[1 0 0]
  Left ear (y) : Integrator  InitialCondition=[0 1 0]
  Matrix Concatenate axes into columns : Concatenate  NumInputs=3  Mode=Multidimensional array  ConcatenateDimension=2
  Position : Integrator  InitialCondition=[0 0 0]
  Scope : Scope
  Sum1 : Sum  Inputs=|++
  Sum2 : Sum  Inputs=|++
  Transpose1 : matrix_library/Transpose
  Transpose2 : matrix_library/Transpose
  Transpose3 : matrix_library/Transpose
  intrinsic to extrinsic : Product  Multiplication=Matrix(*)
  intrinsic to extrinsic1 : Product  Multiplication=Matrix(*)
  Head orientation in world (R xyz in XYZ) : Outport
  Angular velocity (w XYZ) : Outport  Port=2
  Position (p XYZ) : Outport  Port=3
  Velocity (XYZ) : Outport  Port=4
  Acceleration (XYZ) : Outport  Port=5
  wires:
  Head direction (x)/1 -> Scope/1, Matrix Concatenate axes into columns/1, Cross Product4/2
  Cross Product4/1 -> Head direction (x)/1
  Direction rel gravity (z)/1 -> Matrix Concatenate axes into columns/3, Cross Product2/2
  Cross Product2/1 -> Direction rel gravity (z)/1
  Left ear (y)/1 -> Matrix Concatenate axes into columns/2, Cross Product3/2
  Sum1/1 -> Cross Product2/1, Cross Product3/1, Cross Product4/1, Angular velocity (w XYZ)/1
  Cross Product3/1 -> Left ear (y)/1
  Intrinsic velocity (wx wy wz)/1 -> Transpose1/1
  Position/1 -> Position (p XYZ)/1
  Matrix Concatenate axes into columns/1 -> Transpose3/1, Head orientation in world (R xyz in XYZ)/1
  Sum2/1 -> Position/1, Derivative4/1, Velocity (XYZ)/1
  Derivative4/1 -> Acceleration (XYZ)/1
  Extrinsic velocity (wX wY wZ)/1 -> Sum1/1
  Linear extrinsic velocity (vX vY vZ)/1 -> Sum2/1
  Linear intrinsic velocity (vx vy vz)/1 -> Transpose2/1
  intrinsic to extrinsic/1 -> Sum1/2
  intrinsic to extrinsic1/1 -> Sum2/2
  Transpose1/1 -> intrinsic to extrinsic/1
  Transpose2/1 -> intrinsic to extrinsic1/1
  Transpose3/1 -> intrinsic to extrinsic1/2, intrinsic to extrinsic/2

== system OcularMotorLabModel_2023_12_21_M21b/Head velocity (body) ==
  Bus Creator : BusCreator  Tag=Bus Creator  Inputs=3
  FromWs : FromWorkspace  Tag=STV FromWs  VariableName=tuvar
      SigBuilderData=|
      | common.afterFinalStr = 'Extrapolate'
      | common.sampleTime = 0
      | dataSet(1).timeRange = [0 40]
      | dataSet(1).name = 'Zeros'
      | dataSet(2).timeRange = [0 60]
      | dataSet(2).name = 'Sample Sims'
      | sbobj.Groups(1).Name = 'Zeros'
      | sbobj.Groups(1).Signals(1).Name = 'nasooccipital'
      | sbobj.Groups(1).Signals(1).XData = [0 5 6 15 40]
      | sbobj.Groups(1).Signals(1).YData = [0 0 0 0 0]
      | sbobj.Groups(1).Signals(2).Name = 'interaural'
      | sbobj.Groups(1).Signals(2).XData = [0 5 6 40]
      | sbobj.Groups(1).Signals(2).YData = [0 0 0 0]
      | sbobj.Groups(1).Signals(3).Name = 'rostrocaudal'
      | sbobj.Groups(1).Signals(3).XData = [0 5 15 40]
      | sbobj.Groups(1).Signals(3).YData = [0 0 0 0]
      | sbobj.Groups(1).TimeRange = [0 40]
      | sbobj.Groups(2).Name = 'Sample Sims'
      | sbobj.Groups(2).Signals(1).Name = 'nasooccipital'
      | sbobj.Groups(2).Signals(1).XData = [0 5 60]
      | sbobj.Groups(2).Signals(1).YData = [0 0 0]
      | sbobj.Groups(2).Signals(2).Name = 'interaural'
      | sbobj.Groups(2).Signals(2).XData = [0 5 35 60]
      | sbobj.Groups(2).Signals(2).YData = [0 0 0 0]
      | sbobj.Groups(2).Signals(3).Name = 'rostrocaudal'
      | sbobj.Groups(2).Signals(3).XData = [0 20.05 20.05 50.05 50.05 60]
      | sbobj.Groups(2).Signals(3).YData = [0 0 -30 -30 0 0]
      | sbobj.Groups(2).TimeRange = [0 60]
  Subsystem : Subsystem
  Bus : Outport
  wires:
  FromWs/1 -> Subsystem/1(In1)
  Subsystem/1(nasooccipital) -> Bus Creator/1  "nasooccipital"
  Subsystem/2(interaural) -> Bus Creator/2  "interaural"
  Subsystem/3(rostrocaudal) -> Bus Creator/3  "rostrocaudal"
  Bus Creator/1 -> Bus/1

== system OcularMotorLabModel_2023_12_21_M21b/Head velocity (world) ==
  Bus Creator : BusCreator  Tag=Bus Creator  Inputs=3
  FromWs : FromWorkspace  Tag=STV FromWs  VariableName=tuvar
      SigBuilderData=|
      | common.afterFinalStr = 'Extrapolate'
      | common.sampleTime = 0
      | dataSet(1).timeRange = [0 40]
      | dataSet(1).name = 'Zeros'
      | dataSet(2).timeRange = [0 60]
      | dataSet(2).name = 'Sample Sims'
      | dataSet(3).timeRange = [0 40]
      | dataSet(3).name = 'Yaw30degps'
      | dataSet(4).timeRange = [0 40]
      | dataSet(4).name = 'YawHeadImpulse'
      | dataSet(5).timeRange = [0 40]
      | dataSet(5).name = 'PitchHeadImpulse'
      | sbobj.Groups(1).Name = 'Zeros'
      | sbobj.Groups(1).Signals(1).Name = 'x'
      | sbobj.Groups(1).Signals(1).XData = [0 5 6 15 40]
      | sbobj.Groups(1).Signals(1).YData = [0 0 0 0 0]
      | sbobj.Groups(1).Signals(2).Name = 'y'
      | sbobj.Groups(1).Signals(2).XData = [0 5 6 40]
      | sbobj.Groups(1).Signals(2).YData = [0 0 0 0]
      | sbobj.Groups(1).Signals(3).Name = 'z'
      | sbobj.Groups(1).Signals(3).XData = [0 5 15 40]
      | sbobj.Groups(1).Signals(3).YData = [0 0 0 0]
      | sbobj.Groups(1).TimeRange = [0 40]
      | sbobj.Groups(2).Name = 'Sample Sims'
      | sbobj.Groups(2).Signals(1).Name = 'x'
      | sbobj.Groups(2).Signals(1).XData = [0 5 5 10 10 60]
      | sbobj.Groups(2).Signals(1).YData = [0 0 18 18 0 0]
      | sbobj.Groups(2).Signals(2).Name = 'y'
      | sbobj.Groups(2).Signals(2).XData = [0 20.05 50 60]
      | sbobj.Groups(2).Signals(2).YData = [0 0 0 0]
      | sbobj.Groups(2).Signals(3).Name = 'z'
      | sbobj.Groups(2).Signals(3).XData = [0 5 35 60]
      | sbobj.Groups(2).Signals(3).YData = [0 0 0 0]
      | sbobj.Groups(2).TimeRange = [0 60]
      | sbobj.Groups(3).Name = 'Yaw30degps'
      | sbobj.Groups(3).Signals(1).Name = 'x'
      | sbobj.Groups(3).Signals(1).XData = [0 5 6 15 40]
      | sbobj.Groups(3).Signals(1).YData = [0 0 0 0 0]
      | sbobj.Groups(3).Signals(2).Name = 'y'
      | sbobj.Groups(3).Signals(2).XData = [0 5 6 40]
      | sbobj.Groups(3).Signals(2).YData = [0 0 0 0]
      | sbobj.Groups(3).Signals(3).Name = 'z'
      | sbobj.Groups(3).Signals(3).XData = [0 5 5 24.95 24.95 40]
      | sbobj.Groups(3).Signals(3).YData = [0 0 30 30 0 0]
      | sbobj.Groups(3).TimeRange = [0 40]
      | sbobj.Groups(4).Name = 'YawHeadImpulse'
      | sbobj.Groups(4).Signals(1).Name = 'x'
      | sbobj.Groups(4).Signals(1).XData = [0 5 6 15 40]
      | sbobj.Groups(4).Signals(1).YData = [0 0 0 0 0]
      | sbobj.Groups(4).Signals(2).Name = 'y'
      | sbobj.Groups(4).Signals(2).XData = [0 5 6 40]
      | sbobj.Groups(4).Signals(2).YData = [0 0 0 0]
      | sbobj.Groups(4).Signals(3).Name = 'z'
      | sbobj.Groups(4).Signals(3).XData = [0 5 5.1 5.15 5.25 40]
      | sbobj.Groups(4).Signals(3).YData = [0 0 200 200 0 0]
      | sbobj.Groups(4).TimeRange = [0 40]
      | sbobj.Groups(5).Name = 'PitchHeadImpulse'
      | sbobj.Groups(5).Signals(1).Name = 'x'
      | sbobj.Groups(5).Signals(1).XData = [0 5 6 15 40]
      | sbobj.Groups(5).Signals(1).YData = [0 0 0 0 0]
      | sbobj.Groups(5).Signals(2).Name = 'y'
      | sbobj.Groups(5).Signals(2).XData = [0 5.05 5.05 5.25 5.25 40]
      | sbobj.Groups(5).Signals(2).YData = [0 0 300 300 0 0]
      | sbobj.Groups(5).Signals(3).Name = 'z'
      | sbobj.Groups(5).Signals(3).XData = [0 40]
      | sbobj.Groups(5).Signals(3).YData = [0 0]
      | sbobj.Groups(5).TimeRange = [0 40]
  Subsystem : Subsystem
  Bus : Outport
  wires:
  FromWs/1 -> Subsystem/1(In1)
  Subsystem/1(x) -> Bus Creator/1  "x"
  Subsystem/2(y) -> Bus Creator/2  "y"
  Subsystem/3(z) -> Bus Creator/3  "z"
  Bus Creator/1 -> Bus/1

== system OcularMotorLabModel_2023_12_21_M21b/Left eye plant ==
  In1 : Inport
  Demux : Demux  Outputs=3
  Mux : Mux  Inputs=3
  Plant1 : TransferFcn  Numerator=[Tz 1]  Denominator=[T1*T2 (T1+T2) 1]
  Plant2 : TransferFcn  Numerator=[w^2]  Denominator=[1 + 2*psi*w w^2]
  Plant3 : TransferFcn  Numerator=[Tz 1]  Denominator=[T1*T2 (T1+T2) 1]
  Plant4 : TransferFcn  Numerator=[w^2]  Denominator=[1 + 2*psi*w w^2]
  Plant5 : TransferFcn  Numerator=[Tz 1]  Denominator=[T1*T2 (T1+T2) 1]
  Plant6 : TransferFcn  Numerator=[w^2]  Denominator=[1 + 2*psi*w w^2]
  Saturation : Saturate  UpperLimit=50*pi/180  LowerLimit=-50*pi/180
  Eye position : Outport
  wires:
  In1/1 -> Demux/1
  Mux/1 -> Saturation/1  "Eye position"
  Plant4/1 -> Mux/1
  Plant2/1 -> Mux/2
  Plant6/1 -> Mux/3
  Demux/1 -> Plant3/1
  Demux/2 -> Plant1/1
  Demux/3 -> Plant5/1
  Saturation/1 -> Eye position/1
  Plant3/1 -> Plant4/1
  Plant1/1 -> Plant2/1
  Plant5/1 -> Plant6/1

== system OcularMotorLabModel_2023_12_21_M21b/Linear body velocity ==
  Bus Creator : BusCreator  Tag=Bus Creator  Inputs=3
  FromWs : FromWorkspace  Tag=STV FromWs  VariableName=tuvar
      SigBuilderData=|
      | common.afterFinalStr = 'Extrapolate'
      | common.sampleTime = 0
      | dataSet(1).timeRange = [0 40]
      | dataSet(1).name = 'Zeros'
      | dataSet(2).timeRange = [0 60]
      | dataSet(2).name = 'Sample Sims'
      | dataSet(3).timeRange = [0 40]
      | dataSet(3).name = 'Translate forward'
      | sbobj.Groups(1).Name = 'Zeros'
      | sbobj.Groups(1).Signals(1).Name = 'vx'
      | sbobj.Groups(1).Signals(1).XData = [0 5 6 15 40]
      | sbobj.Groups(1).Signals(1).YData = [0 0 0 0 0]
      | sbobj.Groups(1).Signals(2).Name = 'vy'
      | sbobj.Groups(1).Signals(2).XData = [0 5 6 40]
      | sbobj.Groups(1).Signals(2).YData = [0 0 0 0]
      | sbobj.Groups(1).Signals(3).Name = 'vz'
      | sbobj.Groups(1).Signals(3).XData = [0 5 15 40]
      | sbobj.Groups(1).Signals(3).YData = [0 0 0 0]
      | sbobj.Groups(1).TimeRange = [0 40]
      | sbobj.Groups(2).Name = 'Sample Sims'
      | sbobj.Groups(2).Signals(1).Name = 'vx'
      | sbobj.Groups(2).Signals(1).XData = [0 5 60]
      | sbobj.Groups(2).Signals(1).YData = [0 0 0]
      | sbobj.Groups(2).Signals(2).Name = 'vy'
      | sbobj.Groups(2).Signals(2).XData = [0 5 35 60]
      | sbobj.Groups(2).Signals(2).YData = [0 0 0 0]
      | sbobj.Groups(2).Signals(3).Name = 'vz'
      | sbobj.Groups(2).Signals(3).XData = [0 20.05 20.05 50.05 50.05 60]
      | sbobj.Groups(2).Signals(3).YData = [0 0 -30 -30 0 0]
      | sbobj.Groups(2).TimeRange = [0 60]
      | sbobj.Groups(3).Name = 'Translate forward'
      | sbobj.Groups(3).Signals(1).Name = 'vx'
      | sbobj.Groups(3).Signals(1).XData = [0 5 5 6 6 40]
      | sbobj.Groups(3).Signals(1).YData = [0 0 0.81 0.81 0 0]
      | sbobj.Groups(3).Signals(2).Name = 'vy'
      | sbobj.Groups(3).Signals(2).XData = [0 5 6 40]
      | sbobj.Groups(3).Signals(2).YData = [0 0 0 0]
      | sbobj.Groups(3).Signals(3).Name = 'vz'
      | sbobj.Groups(3).Signals(3).XData = [0 5 15 40]
      | sbobj.Groups(3).Signals(3).YData = [0 0 0 0]
      | sbobj.Groups(3).TimeRange = [0 40]
  Subsystem : Subsystem
  Bus : Outport
  wires:
  FromWs/1 -> Subsystem/1(In1)
  Subsystem/1(vx) -> Bus Creator/1  "vx"
  Subsystem/2(vy) -> Bus Creator/2  "vy"
  Subsystem/3(vz) -> Bus Creator/3  "vz"
  Bus Creator/1 -> Bus/1

== system OcularMotorLabModel_2023_12_21_M21b/Linear world velocity ==
  Bus Creator : BusCreator  Tag=Bus Creator  Inputs=3
  FromWs : FromWorkspace  Tag=STV FromWs  VariableName=tuvar
      SigBuilderData=|
      | common.afterFinalStr = 'Extrapolate'
      | common.sampleTime = 0
      | dataSet(1).timeRange = [0 40]
      | dataSet(1).name = 'Zeros'
      | dataSet(2).timeRange = [0 60]
      | dataSet(2).name = 'Sample Sims'
      | dataSet(3).timeRange = [0 40]
      | dataSet(3).name = 'Translate forward'
      | dataSet(4).timeRange = [0 40]
      | dataSet(4).name = 'Translate left'
      | sbobj.Groups(1).Name = 'Zeros'
      | sbobj.Groups(1).Signals(1).Name = 'vX'
      | sbobj.Groups(1).Signals(1).XData = [0 5 6 15 40]
      | sbobj.Groups(1).Signals(1).YData = [0 0 0 0 0]
      | sbobj.Groups(1).Signals(2).Name = 'vY'
      | sbobj.Groups(1).Signals(2).XData = [0 5 6 40]
      | sbobj.Groups(1).Signals(2).YData = [0 0 0 0]
      | sbobj.Groups(1).Signals(3).Name = 'vZ'
      | sbobj.Groups(1).Signals(3).XData = [0 5 15 40]
      | sbobj.Groups(1).Signals(3).YData = [0 0 0 0]
      | sbobj.Groups(1).TimeRange = [0 40]
      | sbobj.Groups(2).Name = 'Sample Sims'
      | sbobj.Groups(2).Signals(1).Name = 'vX'
      | sbobj.Groups(2).Signals(1).XData = [0 5 60]
      | sbobj.Groups(2).Signals(1).YData = [0 0 0]
      | sbobj.Groups(2).Signals(2).Name = 'vY'
      | sbobj.Groups(2).Signals(2).XData = [0 5 35 60]
      | sbobj.Groups(2).Signals(2).YData = [0 0 0 0]
      | sbobj.Groups(2).Signals(3).Name = 'vZ'
      | sbobj.Groups(2).Signals(3).XData = [0 20.05 20.05 50.05 50.05 60]
      | sbobj.Groups(2).Signals(3).YData = [0 0 -30 -30 0 0]
      | sbobj.Groups(2).TimeRange = [0 60]
      | sbobj.Groups(3).Name = 'Translate forward'
      | sbobj.Groups(3).Signals(1).Name = 'vX'
      | sbobj.Groups(3).Signals(1).XData = [0 5 5 6 6 40]
      | sbobj.Groups(3).Signals(1).YData = [0 0 0.81 0.81 0 0]
      | sbobj.Groups(3).Signals(2).Name = 'vY'
      | sbobj.Groups(3).Signals(2).XData = [0 5 6 40]
      | sbobj.Groups(3).Signals(2).YData = [0 0 0 0]
      | sbobj.Groups(3).Signals(3).Name = 'vZ'
      | sbobj.Groups(3).Signals(3).XData = [0 5 15 40]
      | sbobj.Groups(3).Signals(3).YData = [0 0 0 0]
      | sbobj.Groups(3).TimeRange = [0 40]
      | sbobj.Groups(4).Name = 'Translate left'
      | sbobj.Groups(4).Signals(1).Name = 'vX'
      | sbobj.Groups(4).Signals(1).XData = [0 40]
      | sbobj.Groups(4).Signals(1).YData = [0 0]
      | sbobj.Groups(4).Signals(2).Name = 'vY'
      | sbobj.Groups(4).Signals(2).XData = [0 4.5 5 6 6.5 40]
      | sbobj.Groups(4).Signals(2).YData = [0 0 0.3 0.3 0 0]
      | sbobj.Groups(4).Signals(3).Name = 'vZ'
      | sbobj.Groups(4).Signals(3).XData = [0 5 15 40]
      | sbobj.Groups(4).Signals(3).YData = [0 0 0 0]
      | sbobj.Groups(4).TimeRange = [0 40]
  Subsystem : Subsystem
  Bus : Outport
  wires:
  FromWs/1 -> Subsystem/1(In1)
  Subsystem/1(vX) -> Bus Creator/1  "vX"
  Subsystem/2(vY) -> Bus Creator/2  "vY"
  Subsystem/3(vZ) -> Bus Creator/3  "vZ"
  Bus Creator/1 -> Bus/1

== system OcularMotorLabModel_2023_12_21_M21b/Motion TF ==
  note: Symmetric Non linear function that grows linearly up to 50 deg/s (gain of 1) then decreases linearly up to 100 deg/s (gain from 1 gradually to 0) and it's zero after 100 deg/s
      |
      | Aims to simulate how we cannot track visual motion when it is too fast
  In1 : Inport
  Gain5 : Gain  Gain=2
  Saturation2 : Saturate  UpperLimit=50*pi/180  LowerLimit=-50*pi/180
  Saturation3 : Saturate  UpperLimit=100*pi/180  LowerLimit=-100*pi/180
  Sum8 : Sum  Inputs=+|-
  Target velocity : Outport
  wires:
  In1/1 -> Saturation3/1, Saturation2/1
  Saturation2/1 -> Gain5/1
  Saturation3/1 -> Sum8/2
  Gain5/1 -> Sum8/1
  Sum8/1 -> Target velocity/1

== system OcularMotorLabModel_2023_12_21_M21b/Motion TF1 ==
  note: Symmetric Non linear function that grows linearly up to 50 deg/s (gain of 1) then decreases linearly up to 100 deg/s (gain from 1 gradually to 0) and it's zero after 100 deg/s
      |
      | Aims to simulate how we cannot track visual motion when it is too fast
  In1 : Inport
  Gain4 : Gain  Gain=-1
  Gain5 : Gain  Gain=2
  Saturation2 : Saturate  UpperLimit=50*pi/180  LowerLimit=-50*pi/180
  Saturation3 : Saturate  UpperLimit=100*pi/180  LowerLimit=-100*pi/180
  Scope : Scope  NumInputPorts=3
  Sum8 : Sum  Inputs=+|-
  Out1 : Outport
  wires:
  In1/1 -> Gain4/1
  Saturation2/1 -> Gain5/1
  Saturation3/1 -> Scope/2, Sum8/2
  Gain5/1 -> Scope/1, Sum8/1
  Sum8/1 -> Scope/3, Out1/1
  Gain4/1 -> Saturation3/1, Saturation2/1

== system OcularMotorLabModel_2023_12_21_M21b/OCR ==
  EG : Inport
  Asin : Trigonometry  Operator=asin
  DM : Demux  Outputs=3
  Gain7 : Gain  Gain=-0.1
  MX : Mux  Inputs=3
  Out1 : Outport
  wires:
  Asin/1 -> Gain7/1
  Gain7/1 -> MX/1
  EG/1 -> DM/1
  DM/2 -> Asin/1
  MX/1 -> Out1/1

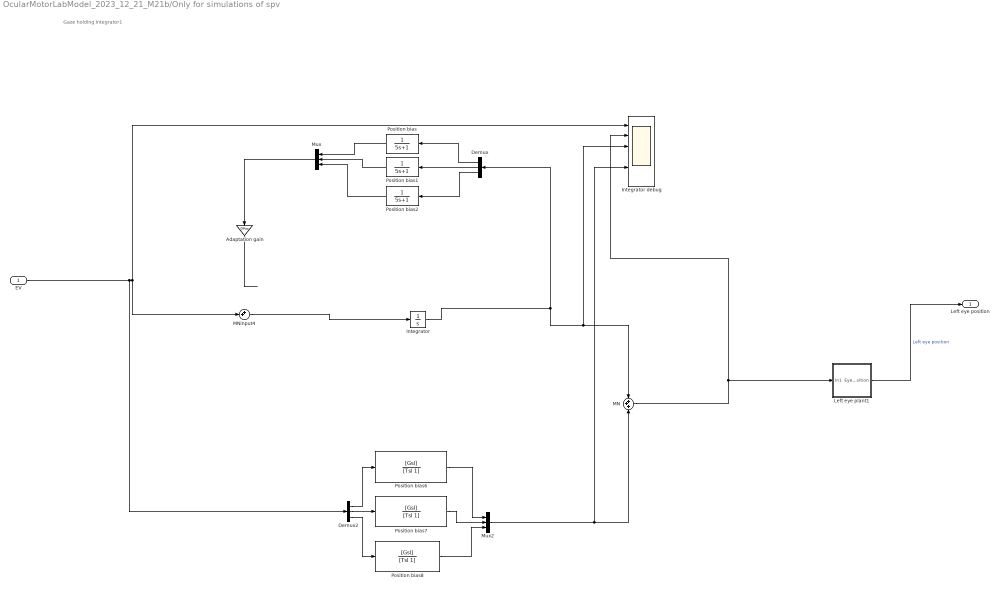
== system OcularMotorLabModel_2023_12_21_M21b/Only for simulations of spv ==
  note: Gaze holding Integrator1
  EV : Inport
  Adaptation gain : Gain  Gain=GPos
  Demux : Demux  Outputs=3
  Demux2 : Demux  Outputs=3
  Integrator : Integrator
  Integrator debug : Scope  NumInputPorts=6
  Left eye plant1 : Subsystem
  "MN " : Sum  Inputs=+++  InputSameDT=on  SaturateOnIntegerOverflow=on  OutDataTypeStr=Inherit: Same as first input
  MNinput4 : Sum  Inputs=++|  InputSameDT=on  SaturateOnIntegerOverflow=on  OutDataTypeStr=Inherit: Same as first input
  Mux : Mux  Inputs=3
  Mux2 : Mux  Inputs=3
  Position bias : TransferFcn  Numerator=1  Denominator=[5 1]
  Position bias1 : TransferFcn  Numerator=1  Denominator=[5 1]
  Position bias2 : TransferFcn  Numerator=1  Denominator=[5 1]
  Position bias6 : TransferFcn  Numerator=[Gsl]  Denominator=[Tsl 1]
  Position bias7 : TransferFcn  Numerator=[Gsl]  Denominator=[Tsl 1]
  Position bias8 : TransferFcn  Numerator=[Gsl]  Denominator=[Tsl 1]
  Left eye position : Outport
  wires:
  "MN "/1 -> Left eye plant1/1(In1), Integrator debug/2
  Left eye plant1/1(Eye position) -> Left eye position/1  "Left eye position"
  Adaptation gain/1 -> ?
  Mux2/1 -> Integrator debug/5, "MN "/3
  Demux2/2 -> Position bias7/1
  Position bias8/1 -> Mux2/3
  Demux2/3 -> Position bias8/1
  Position bias6/1 -> Mux2/1
  Demux2/1 -> Position bias6/1
  EV/1 -> MNinput4/2, Integrator debug/1, Demux2/1
  Position bias7/1 -> Mux2/2
  Integrator/1 -> Integrator debug/3, "MN "/1, Demux/1
  MNinput4/1 -> Integrator/1
  Position bias2/1 -> Mux/3
  Position bias/1 -> Mux/1
  Position bias1/1 -> Mux/2
  Demux/3 -> Position bias2/1
  Demux/2 -> Position bias1/1
  Demux/1 -> Position bias/1
  Mux/1 -> Adaptation gain/1

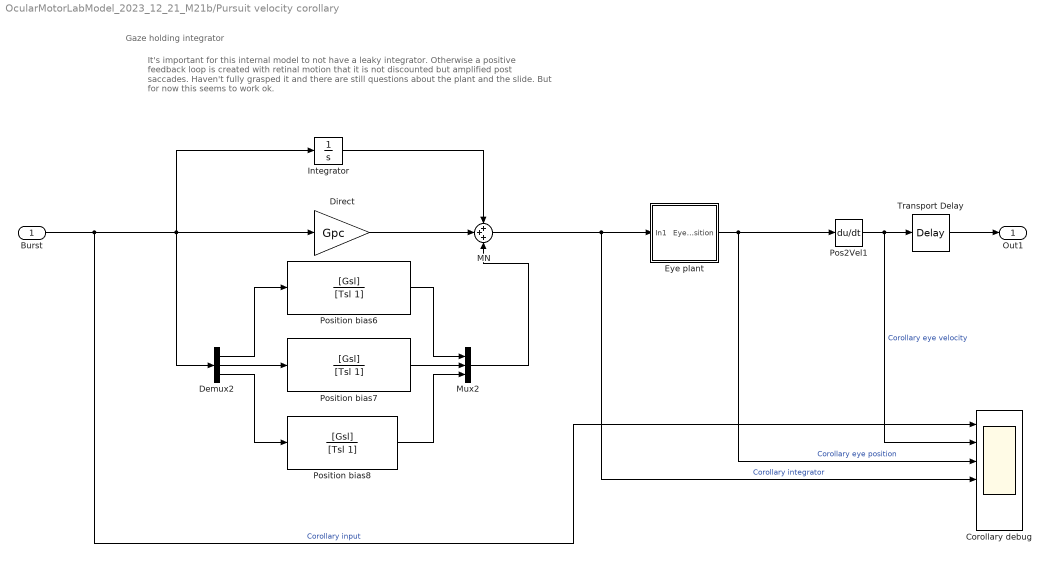
== system OcularMotorLabModel_2023_12_21_M21b/Pursuit velocity corollary ==
  note: Gaze holding integrator
  note: It's important for this internal model to not have a leaky integrator. Otherwise a positive feedback loop is created with retinal motion that it is not discounted but amplified post saccades.
      |
      | Haven't fully grasped it and there are still questions about the plant and the slide. But for now this seems to work ok.
  Burst : Inport
  Corollary debug : Scope  NumInputPorts=6
  Demux2 : Demux  Outputs=3
  Direct : Gain  Gain=Gpc
  Eye plant : Subsystem
  Integrator : Integrator
  "MN " : Sum  Inputs=+++  InputSameDT=on  SaturateOnIntegerOverflow=on  OutDataTypeStr=Inherit: Same as first input
  Mux2 : Mux  Inputs=3
  Pos2Vel1 : Derivative
  Position bias6 : TransferFcn  Numerator=[Gsl]  Denominator=[Tsl 1]
  Position bias7 : TransferFcn  Numerator=[Gsl]  Denominator=[Tsl 1]
  Position bias8 : TransferFcn  Numerator=[Gsl]  Denominator=[Tsl 1]
  Transport Delay : TransportDelay  DelayTime=tdv+tdm
  Out1 : Outport
  wires:
  Burst/1 -> Integrator/1, Direct/1, Demux2/1, Corollary debug/1  "Corollary input"
  Eye plant/1(Eye position) -> Pos2Vel1/1, Corollary debug/3  "Corollary eye position"
  "MN "/1 -> Eye plant/1(In1), Corollary debug/4  "Corollary integrator"
  Transport Delay/1 -> Out1/1
  Pos2Vel1/1 -> Corollary debug/2, Transport Delay/1  "Corollary eye velocity"
  Mux2/1 -> "MN "/3
  Integrator/1 -> "MN "/1
  Demux2/2 -> Position bias7/1
  Position bias8/1 -> Mux2/3
  Demux2/3 -> Position bias8/1
  Position bias6/1 -> Mux2/1
  Demux2/1 -> Position bias6/1
  Position bias7/1 -> Mux2/2
  Direct/1 -> "MN "/2

== system OcularMotorLabModel_2023_12_21_M21b/Right eye plant ==
  In1 : Inport
  Demux : Demux  Outputs=3
  Mux : Mux  Inputs=3
  Plant1 : TransferFcn  Numerator=[Tz 1]  Denominator=[T1*T2 (T1+T2) 1]
  Plant2 : TransferFcn  Numerator=[w^2]  Denominator=[1 + 2*psi*w w^2]
  Plant3 : TransferFcn  Numerator=[Tz 1]  Denominator=[T1*T2 (T1+T2) 1]
  Plant4 : TransferFcn  Numerator=[w^2]  Denominator=[1 + 2*psi*w w^2]
  Plant5 : TransferFcn  Numerator=[Tz 1]  Denominator=[T1*T2 (T1+T2) 1]
  Plant6 : TransferFcn  Numerator=[w^2]  Denominator=[1 + 2*psi*w w^2]
  Saturation : Saturate  UpperLimit=50*pi/180  LowerLimit=-50*pi/180
  Eye position : Outport
  wires:
  In1/1 -> Demux/1
  Mux/1 -> Saturation/1  "Eye position"
  Plant4/1 -> Mux/1
  Plant2/1 -> Mux/2
  Plant6/1 -> Mux/3
  Demux/1 -> Plant3/1
  Demux/2 -> Plant1/1
  Demux/3 -> Plant5/1
  Saturation/1 -> Eye position/1
  Plant3/1 -> Plant4/1
  Plant1/1 -> Plant2/1
  Plant5/1 -> Plant6/1

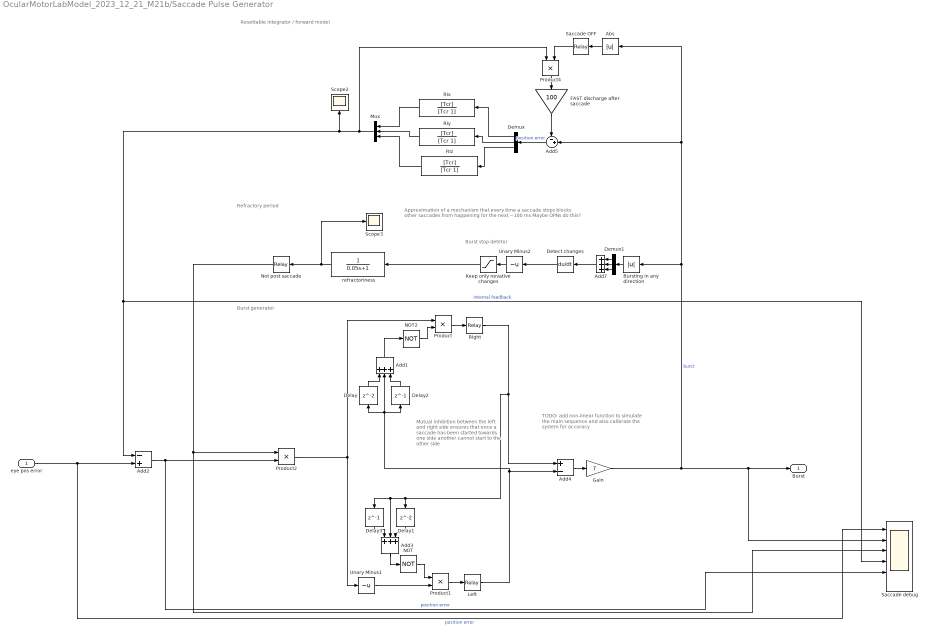
== system OcularMotorLabModel_2023_12_21_M21b/Saccade Pulse Generator ==
  note: Burst generator
  note: Resettable integrator / forward model
  note: Refractory period
  note: Burst stop detetor
  note: Mutual inhibition between the left and right side ensures that once a saccade has been started towards one side another cannot start to the other side
  note: TODO: add non-linear function to simulate the main sequence and also calibrate the system for accuracy
  note: Approximation of a mechanism that every time a saccade stops blocks other saccades from happening for the next ~100 ms
      | Maybe OPNs do this?
  eye pos error : Inport
  Abs : Abs
  Add1 : Sum  Inputs=+++
  Add2 : Sum  Inputs=-+
  Add3 : Sum  Inputs=+++
  Add4 : Sum  Inputs=+-
  Add5 : Sum  Inputs=-+|
  Add7 : Sum  Inputs=+++
  Bursting in any direction : Abs
  Delay : Delay  InitialCondition=0
  Delay1 : Delay  InitialCondition=0
  Delay2 : Delay  DelayLength=1  InitialCondition=0
  Delay3 : Delay  DelayLength=1  InitialCondition=0
  Demux : Demux  Outputs=3
  Demux1 : Demux  Outputs=3
  Detect changes : Derivative
  FAST discharge after saccade : Gain  Gain=100
  Gain : Gain  Gain=7
  Keep only nevative changes : Saturate  UpperLimit=50000000  LowerLimit=0
  Left : Relay  OnSwitchValue=SacThDeg/180*pi  OffSwitchValue=0
  Mux : Mux  Inputs=3
  NOT : Logic  Operator=NOT  IconShape=distinctive  AllPortsSameDT=off  OutDataTypeStr=boolean
  NOT2 : Logic  Operator=NOT  IconShape=distinctive  AllPortsSameDT=off  OutDataTypeStr=boolean
  Not post saccade : Relay  OnSwitchValue=1  OffSwitchValue=1  OnOutputValue=0  OffOutputValue=1
  Product{,1..2,4} (4 alike) : Product
  RIx : TransferFcn  Numerator=[Tcr]  Denominator=[Tcr 1]
  RIy : TransferFcn  Numerator=[Tcr]  Denominator=[Tcr 1]
  RIz : TransferFcn  Numerator=[Tcr]  Denominator=[Tcr 1]
  Right : Relay  OnSwitchValue=SacThDeg/180*pi  OffSwitchValue=0
  Saccade OFF : Relay  OnOutputValue=0  OffOutputValue=1
  Saccade debug : Scope  NumInputPorts=6
  Scope2 : Scope
  Scope3 : Scope
  Unary Minus1 : UnaryMinus
  Unary Minus2 : UnaryMinus
  refractoriness : TransferFcn  Numerator=1  Denominator=[0.05 1]
  Burst : Outport  VectorParamsAs1DForOutWhenUnconnected=off
  wires:
  eye pos error/1 -> Saccade debug/1, Add2/2  "position error"
  Add2/1 -> Saccade debug/5, Product2/2  "position error"
  Add7/1 -> Detect changes/1
  Detect changes/1 -> Unary Minus2/1
  Demux1/1 -> Add7/1
  Demux1/3 -> Add7/3
  Unary Minus2/1 -> Keep only nevative changes/1
  Demux1/2 -> Add7/2
  Bursting in any direction/1 -> Demux1/1
  refractoriness/1 -> Not post saccade/1, Scope3/1
  Keep only nevative changes/1 -> refractoriness/1
  Abs/1 -> Saccade OFF/1
  Product4/1 -> FAST discharge after saccade/1
  Mux/1 -> Saccade debug/4, Add2/1, Scope2/1, Product4/1  "Internal feedback"
  FAST discharge after saccade/1 -> Add5/1
  Saccade OFF/1 -> Product4/2
  Not post saccade/1 -> Saccade debug/3, Product2/1
  Add3/1 -> NOT/1
  Delay/1 -> Add1/1
  Delay2/1 -> Add1/3
  Unary Minus1/1 -> Product1/2
  Add4/1 -> Gain/1
  Product2/1 -> Product/1, Unary Minus1/1
  Add1/1 -> NOT2/1
  Product1/1 -> Left/1
  Product/1 -> Right/1
  NOT2/1 -> Product/2
  Delay1/1 -> Add3/3
  NOT/1 -> Product1/1
  Left/1 -> Add4/2, Delay2/1, Add1/2, Delay/1
  Gain/1 -> Saccade debug/2, Burst/1, Abs/1, Add5/2, Bursting in any direction/1  "burst"
  Delay3/1 -> Add3/1
  Right/1 -> Delay3/1, Add3/2, Delay1/1, Add4/1
  Demux/1 -> RIx/1
  RIy/1 -> Mux/2
  RIx/1 -> Mux/1
  Demux/3 -> RIz/1
  Demux/2 -> RIy/1
  RIz/1 -> Mux/3
  Add5/1 -> Demux/1  "position error"
